simulink subsystem "Drive_d"  (R2022a)
settings: Solver=VariableStepAuto  StartTime=0.0  StopTime=10.0  RelTol=1e-3
settings Model: Creator=12191  LastModifiedBy=12191

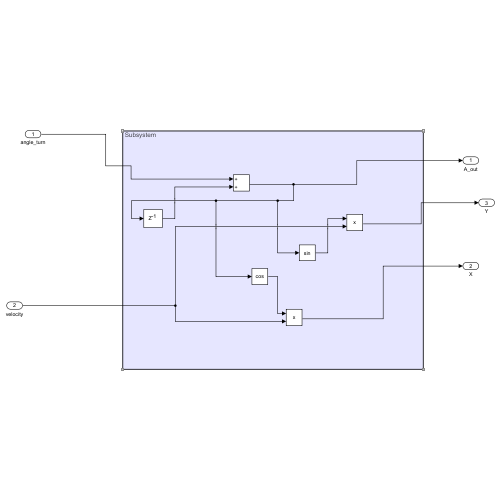
[thumbnail: Simulink's stored preview of the top-level diagram]
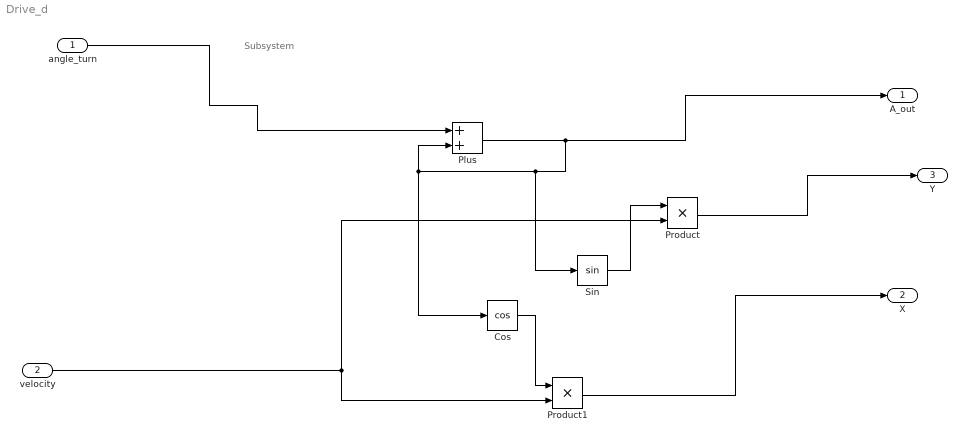
== system Drive_d ==
  note: Subsystem
  angle_turn : Inport
  velocity : Inport  Port=2
  Cos : Trigonometry  Operator=cos
  Plus : Sum
  Product : Product
  Product1 : Product
  Sin : Trigonometry
  A_out : Outport
  X : Outport  Port=2
  Y : Outport  Port=3
  wires:
  angle_turn/1 -> Plus/1
  Plus/1 -> Plus/2, Cos/1, Sin/1, A_out/1
  Sin/1 -> Product/1
  velocity/1 -> Product/2, Product1/2
  Cos/1 -> Product1/1
  Product/1 -> Y/1
  Product1/1 -> X/1
